simulink model "Scenariul1_Raspuns_treapta_sim"  (R2025a)
settings: Solver=ode45  StartTime=0.0  StopTime=5  MaxStep=0.001  RelTol=1e-4
values from neighbouring files (symbols this model uses):
  Kd_PD = 0.5    [Scenariul1_Raspuns_treapta.m]    (also in Scenariul2_Referinta_sinusoidala.m = 0.07; Scenariul3_Sarcina_perturbatoare.m = 0.07)
  Kff = 0.07    [Scenariul1_Raspuns_treapta.m]    (also in Scenariul2_Referinta_sinusoidala.m; Scenariul3_Sarcina_perturbatoare.m = -0.03)
  Ki_PI = 1.5    [Scenariul1_Raspuns_treapta.m]    (also in Scenariul2_Referinta_sinusoidala.m = 0.43; Scenariul3_Sarcina_perturbatoare.m = 7)
  Kp_P = 1.5    [Scenariul1_Raspuns_treapta.m]    (also in Scenariul2_Referinta_sinusoidala.m = 0.35; Scenariul3_Sarcina_perturbatoare.m = 0.36)
  Kp_PD = 1    [Scenariul1_Raspuns_treapta.m]    (also in Scenariul2_Referinta_sinusoidala.m = 3.88; Scenariul3_Sarcina_perturbatoare.m = 3.88)
  Kp_PI = 0.4    [Scenariul1_Raspuns_treapta.m]    (also in Scenariul2_Referinta_sinusoidala.m = 0.11; Scenariul3_Sarcina_perturbatoare.m = 0.7)
settings Model: Creator=luiza  LastModifiedBy=luiza

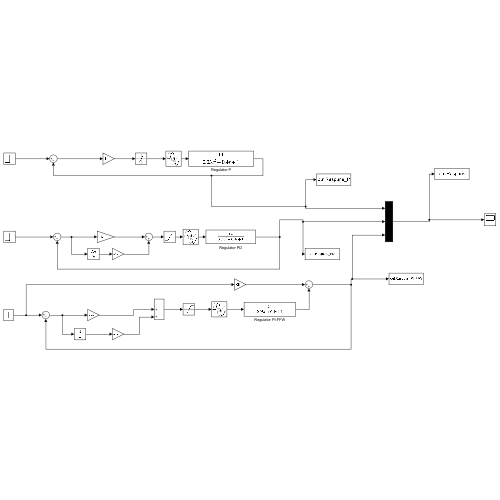
[thumbnail: Simulink's stored preview of the top-level diagram]
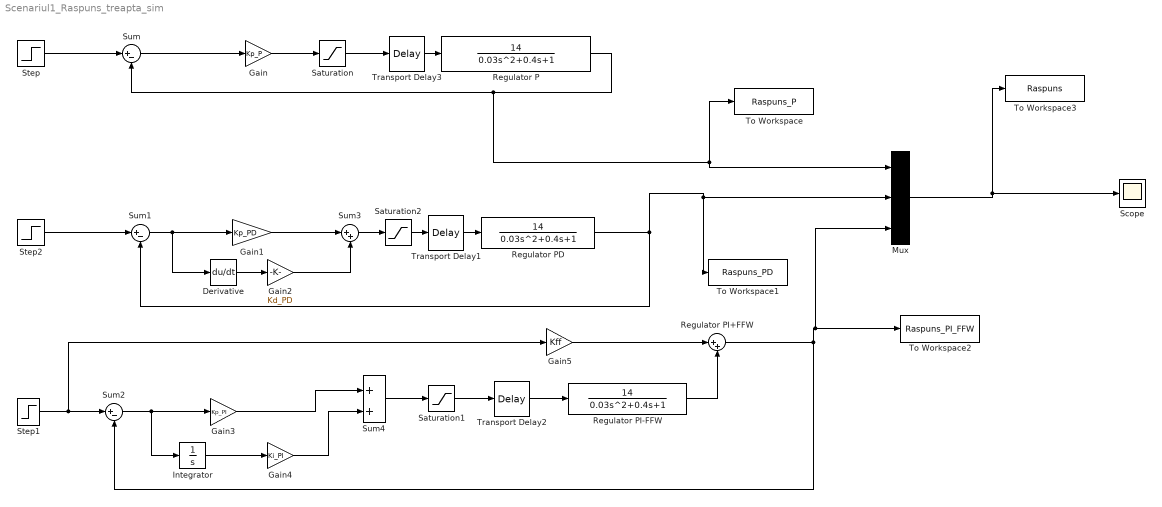
== system Scenariul1_Raspuns_treapta_sim ==
  Derivative : Derivative
  Gain : Gain  Gain=Kp_P
  Gain1 : Gain  Gain=Kp_PD
  Gain2 : Gain  Gain=Kd_PD
  Gain3 : Gain  Gain=Kp_PI
  Gain4 : Gain  Gain=Ki_PI
  Gain5 : Gain  Gain=Kff
  Integrator : Integrator
  Mux : Mux  Inputs=3
  Regulator P : TransferFcn  Numerator=[14]  Denominator=[0.03 0.4 1]
  Regulator PD : TransferFcn  Numerator=[14]  Denominator=[0.03 0.4 1]
  Regulator PI+FFW : Sum  Inputs=|++
  Regulator PI-FFW : TransferFcn  Numerator=[14]  Denominator=[0.03 0.4 1]
  Saturation : Saturate  UpperLimit=100  LowerLimit=-100
  Saturation1 : Saturate  UpperLimit=100  LowerLimit=-100
  Saturation2 : Saturate  UpperLimit=100  LowerLimit=-100
  Scope : Scope
      settings: ActiveDisplayYMinimum=-171.64675581754224  ActiveDisplayYMaximum=189.59726588161504
  Step : Step  Time=0  After=10  SampleTime=0
  Step1 : Step  Time=0  After=10  SampleTime=0
  Step2 : Step  Time=0  After=10  SampleTime=0
  Sum : Sum  Inputs=|+-
  Sum1 : Sum  Inputs=|+-
  Sum2 : Sum  Inputs=|+-
  Sum3 : Sum  Inputs=|++
  Sum4 : Sum  Inputs=|++
  To Workspace : ToWorkspace  VariableName=Raspuns_P  SampleTime=-1
  To Workspace1 : ToWorkspace  VariableName=Raspuns_PD  SampleTime=-1
  To Workspace2 : ToWorkspace  VariableName=Raspuns_PI_FFW  SampleTime=-1
  To Workspace3 : ToWorkspace  VariableName=Raspuns  SampleTime=-1
  Transport Delay1 : TransportDelay  DelayTime=0.05
  Transport Delay2 : TransportDelay  DelayTime=0.05
  Transport Delay3 : TransportDelay  DelayTime=0.05
  wires:
  Step/1 -> Sum/1
  Sum/1 -> Gain/1
  Step2/1 -> Sum1/1
  Sum1/1 -> Derivative/1, Gain1/1
  Derivative/1 -> Gain2/1
  Regulator PD/1 -> Sum1/2, Mux/2, To Workspace1/1
  Step1/1 -> Gain5/1, Sum2/1
  Sum2/1 -> Integrator/1, Gain3/1
  Gain3/1 -> Sum4/1
  Integrator/1 -> Gain4/1
  Gain4/1 -> Sum4/2
  Regulator P/1 -> To Workspace/1, Mux/1, Sum/2
  Mux/1 -> To Workspace3/1, Scope/1
  Gain1/1 -> Sum3/1
  Gain2/1 -> Sum3/2
  Transport Delay1/1 -> Regulator PD/1
  Transport Delay2/1 -> Regulator PI-FFW/1
  Transport Delay3/1 -> Regulator P/1
  Gain/1 -> Saturation/1
  Saturation/1 -> Transport Delay3/1
  Sum3/1 -> Saturation2/1
  Saturation2/1 -> Transport Delay1/1
  Saturation1/1 -> Transport Delay2/1
  Sum4/1 -> Saturation1/1
  Regulator PI-FFW/1 -> Regulator PI+FFW/2
  Gain5/1 -> Regulator PI+FFW/1
  Regulator PI+FFW/1 -> Mux/3, To Workspace2/1, Sum2/2
